simulink model "windTurbulenceS"  (R2019b)
settings: Solver=FixedStepAuto  StartTime=0.0  StopTime=125  FixedStep=0.01  RelTol=1e-3
values from neighbouring files (symbols this model uses):
  DCM = angle2dcm(0, pitch, 0)    [windTurbulence.m]
  h = rE - ((rE^2)/(rE+h))    [getAtmosphereAlt.m]    (also in windTurbulence.m = ry)
  q = 0.5*rho.*vRW.^2    [FlightSim.m]
  r = radius(i)    [FlightSim_distplot.m]    (also in getAtmosphere.m = 7.82620826279e-05)
  V = hypot(vx,vy)    [windTurbulence.m]
undefined symbols (not defined in the file or in its folder): F, Light, MIL, seed
libraries: aerolibwind2 x1
settings Model: EnablePacing=on  PacingRate=1000  Creator=Admin  LastModifiedBy=Admin

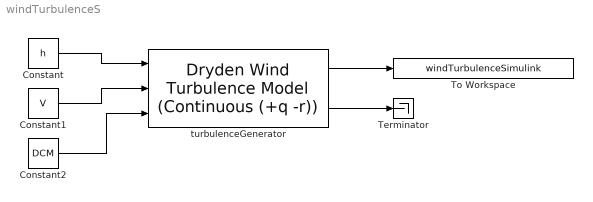
== system windTurbulenceS ==
  Constant : Constant  Value=h
  Constant1 : Constant  Value=V
  Constant2 : Constant  Value=DCM
  Terminator : Terminator
  To Workspace : ToWorkspace  VariableName=windTurbulenceSimulink  SaveFormat=Timeseries  SampleTime=-1
  turbulenceGenerator : aerolibwind2/Dryden Wind Turbulence Model  (Continuous (+q -r))  units=English (Velocity in ft/s)  spec=MIL-F-8785C  model=Continuous Von Karman (+q +r)  W20=meanWind  Wdeg=0  TurbProb=10^-2 - Light  L_high=762  Wingspan=2  ts=0.01  Seed=seed  T_on=on
      settings: SourceProductName=Aerospace Blockset
  wires:
  turbulenceGenerator/1 -> To Workspace/1
  Constant/1 -> turbulenceGenerator/1
  Constant1/1 -> turbulenceGenerator/2
  Constant2/1 -> turbulenceGenerator/3
  turbulenceGenerator/2 -> Terminator/1
